simulink model "Inverted_pendulum"  (R2019b)
settings: Solver=VariableStepAuto  StartTime=0.0  StopTime=5  RelTol=1e-3
values from neighbouring files (symbols this model uses):
  b = 0.1    [laplace_model.m]
  g = 9.8    [laplace_model.m]
  I = 0.006    [laplace_model.m]
  l = 0.3    [laplace_model.m]
  m = 0.2    [laplace_model.m]
  M = 0.5    [laplace_model.m]
  q = (M+m)*(I+m*l^2)-(m*l)^2    (= 0.0132)    [laplace_model.m]
settings Model: Creator=prateekm  LastModifiedBy=BHUSHAN
settings SFSimCC: CustomCodeUndefinedFunction=UseInterfaceOnly

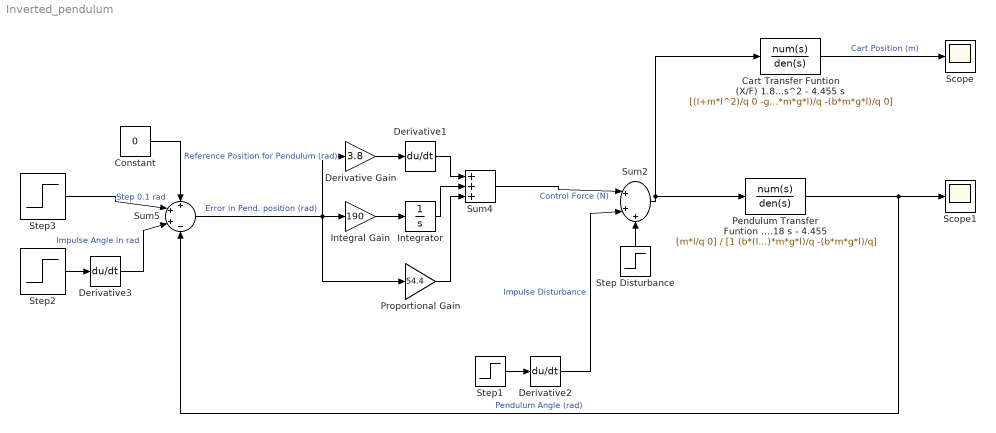
== system Inverted_pendulum ==
  "Cart Transfer Funtion (X/F) 1.818 s^2 - 44.55 -------------------------------------- s^4 + 0.1818 s^3 - 31.18 s^2 - 4.455 s " : TransferFcn  Numerator=[(I+m*l^2)/q 0 -g*m*l/q]  Denominator=[1 (b*(I+m*l^2))/q -((M+m)*m*g*l)/q -(b*m*g*l)/q 0]
  Constant : Constant  Value=0
  Derivative Gain : Gain  Gain=3.8
  Derivative1 : Derivative
  Derivative2 : Derivative
  Derivative3 : Derivative
  Integral Gain : Gain  Gain=190
  "Integrator " : Integrator
  Pendulum Transfer Funtion 4.545 s ---------------------------------- s^3 + 0.1818 s^2 - 31.18 s - 4.455 : TransferFcn  Numerator=[m*l/q 0]  Denominator=[1 (b*(I+m*l^2))/q -((M+m)*m*g*l)/q -(b*m*g*l)/q]
  Proportional Gain : Gain  Gain=54.4
  Scope : Scope
  Scope1 : Scope
  Step Disturbance : Step  Time=0  After=0  SampleTime=0
  Step1 : Step  Time=0  After=0  SampleTime=0
  Step2 : Step  Time=0  After=0  SampleTime=0
  Step3 : Step  Time=0  After=0  SampleTime=0
  Sum2 : Sum  Inputs=|+++
  Sum4 : Sum  Inputs=+++
  Sum5 : Sum  Inputs=+++-
  wires:
  Constant/1 -> Sum5/1  "Reference Position for Pendulum (rad)"
  Pendulum Transfer Funtion 4.545 s ---------------------------------- s^3 + 0.1818 s^2 - 31.18 s - 4.455/1 -> Sum5/4, Scope1/1  "Pendulum Angle (rad)"
  Integral Gain/1 -> "Integrator "/1
  Derivative Gain/1 -> Derivative1/1
  Sum2/1 -> "Cart Transfer Funtion (X/F) 1.818 s^2 - 44.55 -------------------------------------- s^4 + 0.1818 s^3 - 31.18 s^2 - 4.455 s "/1, Pendulum Transfer Funtion 4.545 s ---------------------------------- s^3 + 0.1818 s^2 - 31.18 s - 4.455/1
  "Integrator "/1 -> Sum4/2
  Derivative1/1 -> Sum4/1
  Sum4/1 -> Sum2/1  "Control Force (N)"
  Proportional Gain/1 -> Sum4/3
  Step1/1 -> Derivative2/1
  "Cart Transfer Funtion (X/F) 1.818 s^2 - 44.55 -------------------------------------- s^4 + 0.1818 s^3 - 31.18 s^2 - 4.455 s "/1 -> Scope/1  "Cart Position (m)"
  Sum5/1 -> Proportional Gain/1, Integral Gain/1, Derivative Gain/1  "Error in Pend. position (rad)"
  Step Disturbance/1 -> Sum2/3
  Step2/1 -> Derivative3/1
  Derivative2/1 -> Sum2/2  "Impulse Disturbance"
  Derivative3/1 -> Sum5/3  "Impulse Angle in rad"
  Step3/1 -> Sum5/2  "Step 0.1 rad"
